simulink model "ES101A_DiagcMgr"  (R2013b)
settings: Solver=ode45  StartTime=0.0  StopTime=0.44  RelTol=1e-3
values from neighbouring files (symbols this model uses):
  BrdgVltg = DataDict.IpSignal    [ES101A_DiagcMgr_DataDict.m]
  DEM_CLEAR_PENDING = DataDict.Constant    [ES101A_DiagcMgr_DataDict.m]
  DEM_DTC_GROUP_ALL_DTCS = DataDict.Constant    [ES101A_DiagcMgr_DataDict.m]
  DFTAGICNTR_CNT_U08 = DataDict.Constant    [ES101A_DiagcMgr_DataDict.m]
  DIAGCMGR_NTCINFOSTSTESTFAILD_CNT_U08 = DataDict.Constant    [ES101A_DiagcMgr_DataDict.m]
  DIAGCMGR_NTCINFOSTSTESTFAILDTHISIGNCYC_CNT_U08 = DataDict.Constant    [ES101A_DiagcMgr_DataDict.m]
  DIAGCMGR_NTCINFOSTSTESTNOTCMPLTHISIGNCYC_CNT_U08 = DataDict.Constant    [ES101A_DiagcMgr_DataDict.m]
  DiagcMgrFltResp = DataDict.Calibration    [ES101A_DiagcMgr_DataDict.m]
  DiagcMgrNtcFltAry = DataDict.NVM    [ES101A_DiagcMgr_DataDict.m]
  DIAGCSTSCTRLDSHTDWNFLTPRSNT_CNT_U16 = DataDict.Constant    [ES101A_DiagcMgr_DataDict.m]
  DIAGCSTSDFTHWAG_CNT_U16 = DataDict.Constant    [ES101A_DiagcMgr_DataDict.m]
  DIAGCSTSDFTHWAGSERLCOMEXPRTVAL_CNT_U16 = DataDict.Constant    [ES101A_DiagcMgr_DataDict.m]
  DIAGCSTSDFTVEHSPD_CNT_U16 = DataDict.Constant    [ES101A_DiagcMgr_DataDict.m]
  DIAGCSTSININVAL_CNT_U16 = DataDict.Constant    [ES101A_DiagcMgr_DataDict.m]
  DIAGCSTSIVTR1INACTV_CNT_U16 = DataDict.Constant    [ES101A_DiagcMgr_DataDict.m]
  DIAGCSTSIVTR2INACTV_CNT_U16 = DataDict.Constant    [ES101A_DiagcMgr_DataDict.m]
  DIAGCSTSLIMDTPRFMNC_CNT_U16 = DataDict.Constant    [ES101A_DiagcMgr_DataDict.m]
  DIAGCSTSRAMPTOZEROFLTPRSNT_CNT_U16 = DataDict.Constant    [ES101A_DiagcMgr_DataDict.m]
  DIAGCSTSWHLIMBREJCTNDI_CNT_U16 = DataDict.Constant    [ES101A_DiagcMgr_DataDict.m]
  DTCIDXSTSFAIL_CNT_U08 = DataDict.Constant    [ES101A_DiagcMgr_DataDict.m]
  DTCIDXSTSNONTC_CNT_U08 = DataDict.Constant    [ES101A_DiagcMgr_DataDict.m]
  DTCIDXSTSNORES_CNT_U08 = DataDict.Constant    [ES101A_DiagcMgr_DataDict.m]
  DTCIDXSTSPASS_CNT_U08 = DataDict.Constant    [ES101A_DiagcMgr_DataDict.m]
  DTCIDXSTSUPDCFMD_CNT_U08 = DataDict.Constant    [ES101A_DiagcMgr_DataDict.m]
  ELECGLBPRM_IVTRCNT_CNT_U08 = DataDict.ConfigParam    [ES101A_DiagcMgr_DataDict.m]
  FLTINJ_DIAGCMGR_DIAGCSTSIVTR1INACTV = DataDict.Constant    [ES101A_DiagcMgr_DataDict.m]
  FLTINJ_DIAGCMGR_DIAGCSTSIVTR2INACTV = DataDict.Constant    [ES101A_DiagcMgr_DataDict.m]
  HwTq = DataDict.IpSignal    [ES101A_DiagcMgr_DataDict.m]
  IgnCntr = DataDict.IpSignal    [ES101A_DiagcMgr_DataDict.m]
  MAXDEBCNTRVAL_CNT_S16 = DataDict.Constant    [ES101A_DiagcMgr_DataDict.m]
  MAXRAMPRATE_ULSPERSEC_F32 = DataDict.Constant    [ES101A_DiagcMgr_DataDict.m]
  MINDEBCNTRVAL_CNT_S16 = DataDict.Constant    [ES101A_DiagcMgr_DataDict.m]
  MINRAMPRATE_ULSPERSEC_F32 = DataDict.Constant    [ES101A_DiagcMgr_DataDict.m]
  SCAMOTTQCMDTOONE_ULS_F32 = DataDict.Constant    [ES101A_DiagcMgr_DataDict.m]
  SCAMOTTQCMDTOZERO_ULS_F32 = DataDict.Constant    [ES101A_DiagcMgr_DataDict.m]
  SysSt = DataDict.IpSignal    [ES101A_DiagcMgr_DataDict.m]
  VehSpd = DataDict.IpSignal    [ES101A_DiagcMgr_DataDict.m]
undefined symbols (not defined in the file or in its folder): ActvMotTqCmdSca, ActvRampRate, AgiCntr, Dem_DTCFormatType, Dem_DTCOriginType, Dem_EventStatusType, DiagcData, DiagcMgrNtcMap, DiagcSts, DtcEnaMask, EcuT, HistNtcFltAry, MicroDiagcData, MotTq, NtcNr, NtcNrWithResd1, NtcStInfo, ProxySetNtcData, Sts, SysSt1, TOTNROFDTC_CNT_U08
libraries: simulink x151, FloatToFixd x5, NxtrNvM x4
(part 3 of 13)

== system ES101A_DiagcMgr/DiagcMgr/ClrAllDiagc/If Action Subsystem1 ==
  Action Port : ActionPort  ActionType=else
  Set : Constant
  ClrDiagcFlg : Outport
  wires:
  Set/1 -> ClrDiagcFlg/1

== system ES101A_DiagcMgr/DiagcMgr/ClrSnpshtData/CopyRight2 ==

== system ES101A_DiagcMgr/DiagcMgr/ClrSnpshtData/Subsystem ==
  Length of Snapshot Array : Inport
  Assignment1 : Assignment  IndexMode=Zero-based  IndexOptions=Index vector (port)  Indices=1  OutputSizes=1
  Bus Assignment3 : BusAssignment  AssignedSignals=MicroDiagcData,HwTq,MotTq,IgnCntr,BrdgVltg,EcuT,NtcNr,NtcStInfo,SysSt,VehSpd
  Constant1 : Constant  Value=0  OutDataTypeStr=uint32
  Constant12 : Constant  Value=0  OutDataTypeStr=uint8
  Constant{2..4,7..8} (5 alike) : Constant  Value=0  OutDataTypeStr=single
  Constant5 : Constant  Value=SysSt1.SYSST_WRMININ  OutDataTypeStr=Enum: SysSt1
  Constant6 : Constant  Value=0  OutDataTypeStr=uint32
  Constant9 : Constant  Value=NtcNrWithResd1.NTCNR_RESD  OutDataTypeStr=Enum: NtcNrWithResd1
  CopyRight2 : Subsystem  Description=|  mask(Copyright Information){none=on}
      | Copyright info block.                                               
      |                                                                     
      | Place copyright information at the top of every subsystem in design.
      mask prompts: none "No parameters"
      mask help: Place copyright information at the top of every subsystem in design.
      mask Display:
      | NxtrConf = 'Nexteer Confidential';
      | 
      | sys = bdroot; %handle for the current model ("system")
      | first = get_param(sys,'Created');
      | first = first(end-3:end);  %year is last four digits
      | 
      | last = get_param(sys,'LastModifiedDate');
      | if isempty(last)
      |     last = datestr(now,'yyyy');
      | else
      |     last = last(end-3:end);
      | end
      | 
      | if strcmp(first,last)
      |     fprintf('%s -- Copyright %s Nexteer',NxtrConf,first)
      | else
      |     fprintf('%s -- %s%s- %s Nexteer',NxtrConf,char(169),first,last)
      | end
  Data Store Read1 : DataStoreRead  DataStoreName=SnpshtDataAry
  Data Store Write2 : DataStoreWrite  DataStoreName=SnpshtDataAry
  For Iterator : ForIterator  IterationSource=external  IndexMode=Zero-based
  Selector1 : Selector  IndexMode=Zero-based  InputPortWidth=20  IndexOptions=Index vector (port)  Indices=[1 3]  OutputSizes=1
  wires:
  Length of Snapshot Array/1 -> For Iterator/1
  For Iterator/1 -> Selector1/2, Assignment1/3
  Bus Assignment3/1 -> Assignment1/2
  Assignment1/1 -> Data Store Write2/1
  Selector1/1 -> Bus Assignment3/1
  Data Store Read1/1 -> Selector1/1, Assignment1/1
  Constant9/1 -> Bus Assignment3/8
  Constant5/1 -> Bus Assignment3/10
  Constant12/1 -> Bus Assignment3/9
  Constant6/1 -> Bus Assignment3/5
  Constant3/1 -> Bus Assignment3/4
  Constant2/1 -> Bus Assignment3/3
  Constant4/1 -> Bus Assignment3/11
  Constant8/1 -> Bus Assignment3/7
  Constant1/1 -> Bus Assignment3/2
  Constant7/1 -> Bus Assignment3/6

== system ES101A_DiagcMgr/DiagcMgr/DiagcMgrIninCore/CopyRight2 ==

== system ES101A_DiagcMgr/DiagcMgr/DiagcMgrIninCore/Initialize the NtcInfo Array ==
  NtcInfoArySize : Inport
  NtcInfoAry_ArgIn : Inport  Port=2
  CopyRight2 : Subsystem  Description=|  mask(Copyright Information){none=on}
      | Copyright info block.                                               
      |                                                                     
      | Place copyright information at the top of every subsystem in design.
      mask prompts: none "No parameters"
      mask help: Place copyright information at the top of every subsystem in design.
      mask Display:
      | NxtrConf = 'Nexteer Confidential';
      | 
      | sys = bdroot; %handle for the current model ("system")
      | first = get_param(sys,'Created');
      | first = first(end-3:end);  %year is last four digits
      | 
      | last = get_param(sys,'LastModifiedDate');
      | if isempty(last)
      |     last = datestr(now,'yyyy');
      | else
      |     last = last(end-3:end);
      | end
      | 
      | if strcmp(first,last)
      |     fprintf('%s -- Copyright %s Nexteer',NxtrConf,first)
      | else
      |     fprintf('%s -- %s%s- %s Nexteer',NxtrConf,char(169),first,last)
      | end
  Update the ISO bits of each NTC : Subsystem  RequirementInfo={} %GIDa_598903a9_4093_4047_8f55_d30b0bb8de3e  Priority=2  TreatAsAtomicUnit=on
      settings: AttributesFormatString=Priority = %<Priority>
  NtcInfoAry_ArgOut : Outport
  wires:
  NtcInfoArySize/1 -> Update the ISO bits of each NTC/1(Number of Iteration)
  Update the ISO bits of each NTC/1(NtcInfoAry_ArgOut) -> NtcInfoAry_ArgOut/1
  NtcInfoAry_ArgIn/1 -> Update the ISO bits of each NTC/2(NtcInfoAry_ArgIn)

== system ES101A_DiagcMgr/DiagcMgr/DiagcMgrIninCore/Update DiagcSts and DiagcMgrActv ==
  note: ProxySetNtcData and DiagcData are inputs to the port "Bus"
      | of the Bus Assignment Block are not inputs, outputs or arguments to the
      | DiagcMgrIninCore. They are being used for modelling purpose to show
      | that the data is being written to the respective structs.
  ProxySetNtcData : Inport
  DiagcData : Inport  Port=2
  Bus Assignment1 : BusAssignment  AssignedSignals=DiagcSts,ActvRampRate,ActvMotTqCmdSca
  Bus Assignment2 : BusAssignment  AssignedSignals=DiagcSts,ActvRampRate,ActvMotTqCmdSca
  CopyRight2 : Subsystem  Description=|  mask(Copyright Information){none=on}
      | Copyright info block.                                               
      |                                                                     
      | Place copyright information at the top of every subsystem in design.
      mask prompts: none "No parameters"
      mask help: Place copyright information at the top of every subsystem in design.
      mask Display:
      | NxtrConf = 'Nexteer Confidential';
      | 
      | sys = bdroot; %handle for the current model ("system")
      | first = get_param(sys,'Created');
      | first = first(end-3:end);  %year is last four digits
      | 
      | last = get_param(sys,'LastModifiedDate');
      | if isempty(last)
      |     last = datestr(now,'yyyy');
      | else
      |     last = last(end-3:end);
      | end
      | 
      | if strcmp(first,last)
      |     fprintf('%s -- Copyright %s Nexteer',NxtrConf,first)
      | else
      |     fprintf('%s -- %s%s- %s Nexteer',NxtrConf,char(169),first,last)
      | end
  DiagcStsActvMotTqCmdSca : Constant  Value=SCAMOTTQCMDTOONE_ULS_F32  OutDataTypeStr=single
  DiagcStsActvRampRate : Constant  Value=MINRAMPRATE_ULSPERSEC_F32  OutDataTypeStr=single
  Dual Inverter : Subsystem  TreatAsAtomicUnit=on
  If1 : If  IfExpression=u1 == 1
  Merge : Merge
  Number of Inverters : Constant  Value=ELECGLBPRM_IVTRCNT_CNT_U08
  ProxySetNtcActvMotTqCmdSca : Constant  Value=SCAMOTTQCMDTOONE_ULS_F32  OutDataTypeStr=single
  ProxySetNtcActvRampRate : Constant  Value=MINRAMPRATE_ULSPERSEC_F32  OutDataTypeStr=single
  Single Inverter : Subsystem  Description=""  TreatAsAtomicUnit=on
      settings: AttributesFormatString=%<Description>
  ProxySetNtcData_ArgOut : Outport
  DiagcData_ArgOut : Outport  Port=2
  wires:
  Number of Inverters/1 -> If1/1
  If1/1 -> Single Inverter/Action
  ProxySetNtcActvMotTqCmdSca/1 -> Bus Assignment1/4
  ProxySetNtcActvRampRate/1 -> Bus Assignment1/3
  Bus Assignment1/1 -> ProxySetNtcData_ArgOut/1
  If1/2 -> Dual Inverter/Action
  Single Inverter/1(DiagcSts) -> Merge/1
  Dual Inverter/1(DiagcSts) -> Merge/2
  Merge/1 -> Bus Assignment2/2, Bus Assignment1/2
  Bus Assignment2/1 -> DiagcData_ArgOut/1
  DiagcStsActvRampRate/1 -> Bus Assignment2/3
  DiagcStsActvMotTqCmdSca/1 -> Bus Assignment2/4
  ProxySetNtcData/1 -> Bus Assignment1/1
  DiagcData/1 -> Bus Assignment2/1

== system ES101A_DiagcMgr/DiagcMgr/DiagcMgrIninCore/Update NtcInfoAry From NvM ==
  AppIdx_ArgIn : Inport
  NtcInfoAry_ArgIn : Inport  Port=2
  CopyRight2 : Subsystem  Description=|  mask(Copyright Information){none=on}
      | Copyright info block.                                               
      |                                                                     
      | Place copyright information at the top of every subsystem in design.
      mask prompts: none "No parameters"
      mask help: Place copyright information at the top of every subsystem in design.
      mask Display:
      | NxtrConf = 'Nexteer Confidential';
      | 
      | sys = bdroot; %handle for the current model ("system")
      | first = get_param(sys,'Created');
      | first = first(end-3:end);  %year is last four digits
      | 
      | last = get_param(sys,'LastModifiedDate');
      | if isempty(last)
      |     last = datestr(now,'yyyy');
      | else
      |     last = last(end-3:end);
      | end
      | 
      | if strcmp(first,last)
      |     fprintf('%s -- Copyright %s Nexteer',NxtrConf,first)
      | else
      |     fprintf('%s -- %s%s- %s Nexteer',NxtrConf,char(169),first,last)
      | end
  Data Store Read1 : DataStoreRead  DataStoreName=DiagcMgrNtcFltAry
  Update NtcInfoAry : Subsystem
  Width : Width  DataType=uint8
  NtcInfoAry_ArgOut : Outport
  wires:
  Width/1 -> Update NtcInfoAry/1(Length of NtcFltArray)
  AppIdx_ArgIn/1 -> Update NtcInfoAry/2(AppIdx_ArgIn)
  Data Store Read1/1 -> Width/1
  NtcInfoAry_ArgIn/1 -> Update NtcInfoAry/3(NtcInfoAry_ArgIn)
  Update NtcInfoAry/1(NtcInfoAry_ArgOut) -> NtcInfoAry_ArgOut/1

== system ES101A_DiagcMgr/DiagcMgr/DiagcMgrPer1/CopyRight2 ==

== system ES101A_DiagcMgr/DiagcMgr/DiagcMgrPer1/Update OutpDiagcData ==
  Bus Selector : BusSelector  OutputSignals=DiagcSts,ActvRampRate,ActvMotTqCmdSca
  CopyRight2 : Subsystem  Description=|  mask(Copyright Information){none=on}
      | Copyright info block.                                               
      |                                                                     
      | Place copyright information at the top of every subsystem in design.
      mask prompts: none "No parameters"
      mask help: Place copyright information at the top of every subsystem in design.
      mask Display:
      | NxtrConf = 'Nexteer Confidential';
      | 
      | sys = bdroot; %handle for the current model ("system")
      | first = get_param(sys,'Created');
      | first = first(end-3:end);  %year is last four digits
      | 
      | last = get_param(sys,'LastModifiedDate');
      | if isempty(last)
      |     last = datestr(now,'yyyy');
      | else
      |     last = last(end-3:end);
      | end
      | 
      | if strcmp(first,last)
      |     fprintf('%s -- Copyright %s Nexteer',NxtrConf,first)
      | else
      |     fprintf('%s -- %s%s- %s Nexteer',NxtrConf,char(169),first,last)
      | end
  GetDiagcDataApplX : Subsystem  RequirementInfo={} %GIDa_c222c484_d216_46ea_ad62_3550c5adb482
      settings: AttributesFormatString=%<Description>
  OutpDiagcSts : Outport
  OutpRampRate : Outport  Port=2
  OutpMotTqCmdSca : Outport  Port=3
  wires:
  Bus Selector/1 -> OutpDiagcSts/1  "<DiagcSts>"
  Bus Selector/3 -> OutpMotTqCmdSca/1  "<ActvMotTqCmdSca>"
  Bus Selector/2 -> OutpRampRate/1  "<ActvRampRate>"
  GetDiagcDataApplX/1(TempDiagcData) -> Bus Selector/1

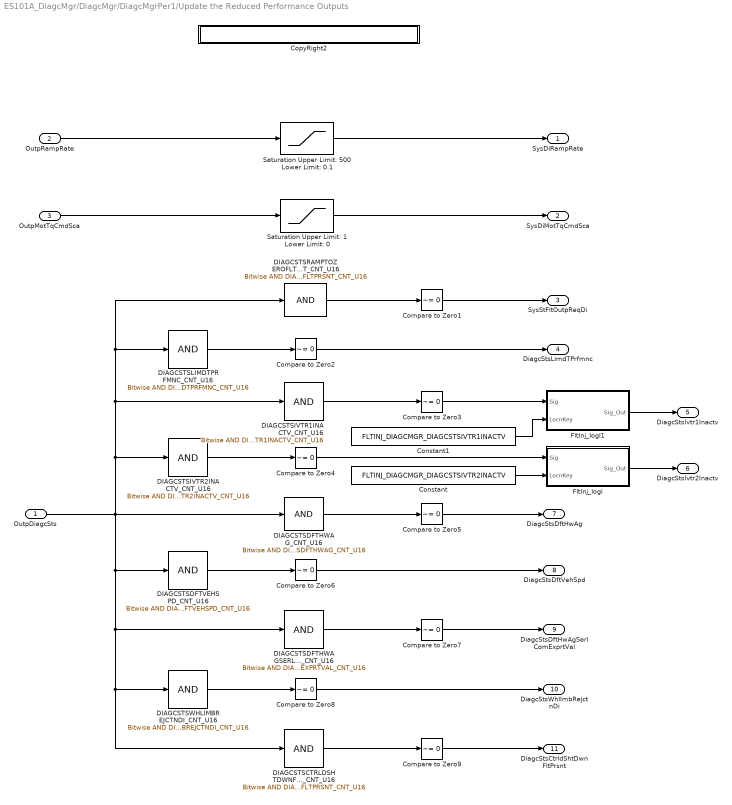
== system ES101A_DiagcMgr/DiagcMgr/DiagcMgrPer1/Update the Reduced Performance Outputs ==
  OutpDiagcSts : Inport
  OutpRampRate : Inport  Port=2
  OutpMotTqCmdSca : Inport  Port=3
  Compare to Zero{1..9} (9 alike) : simulink/Logic and Bit Operations/Compare To Zero  relop=~=  OutDataTypeStr=boolean
  Constant : Constant  Value=FLTINJ_DIAGCMGR_DIAGCSTSIVTR2INACTV
  Constant1 : Constant  Value=FLTINJ_DIAGCMGR_DIAGCSTSIVTR1INACTV
  CopyRight2 : Subsystem  Description=|  mask(Copyright Information){none=on}
      | Copyright info block.                                               
      |                                                                     
      | Place copyright information at the top of every subsystem in design.
      mask prompts: none "No parameters"
      mask help: Place copyright information at the top of every subsystem in design.
      mask Display:
      | NxtrConf = 'Nexteer Confidential';
      | 
      | sys = bdroot; %handle for the current model ("system")
      | first = get_param(sys,'Created');
      | first = first(end-3:end);  %year is last four digits
      | 
      | last = get_param(sys,'LastModifiedDate');
      | if isempty(last)
      |     last = datestr(now,'yyyy');
      | else
      |     last = last(end-3:end);
      | end
      | 
      | if strcmp(first,last)
      |     fprintf('%s -- Copyright %s Nexteer',NxtrConf,first)
      | else
      |     fprintf('%s -- %s%s- %s Nexteer',NxtrConf,char(169),first,last)
      | end
  DIAGCSTSCTRLDSHTDWNFLTPRSNT_CNT_U16 : simulink/Logic and Bit Operations/Bitwise Operator  logicop=AND  UseBitMask=on  BitMask=DIAGCSTSCTRLDSHTDWNFLTPRSNT_CNT_U16  BitMaskRealWorld=Stored Integer
  DIAGCSTSDFTHWAGSERLCOMEXPRTVAL_CNT_U16 : simulink/Logic and Bit Operations/Bitwise Operator  logicop=AND  UseBitMask=on  BitMask=DIAGCSTSDFTHWAGSERLCOMEXPRTVAL_CNT_U16  BitMaskRealWorld=Stored Integer
  DIAGCSTSDFTHWAG_CNT_U16 : simulink/Logic and Bit Operations/Bitwise Operator  logicop=AND  UseBitMask=on  BitMask=DIAGCSTSDFTHWAG_CNT_U16  BitMaskRealWorld=Stored Integer
  DIAGCSTSDFTVEHSPD_CNT_U16 : simulink/Logic and Bit Operations/Bitwise Operator  logicop=AND  UseBitMask=on  BitMask=DIAGCSTSDFTVEHSPD_CNT_U16  BitMaskRealWorld=Stored Integer
  DIAGCSTSIVTR1INACTV_CNT_U16 : simulink/Logic and Bit Operations/Bitwise Operator  logicop=AND  UseBitMask=on  BitMask=DIAGCSTSIVTR1INACTV_CNT_U16  BitMaskRealWorld=Stored Integer
  DIAGCSTSIVTR2INACTV_CNT_U16 : simulink/Logic and Bit Operations/Bitwise Operator  logicop=AND  UseBitMask=on  BitMask=DIAGCSTSIVTR2INACTV_CNT_U16  BitMaskRealWorld=Stored Integer
  DIAGCSTSLIMDTPRFMNC_CNT_U16 : simulink/Logic and Bit Operations/Bitwise Operator  logicop=AND  UseBitMask=on  BitMask=DIAGCSTSLIMDTPRFMNC_CNT_U16  BitMaskRealWorld=Stored Integer
  DIAGCSTSRAMPTOZEROFLTPRSNT_CNT_U16 : simulink/Logic and Bit Operations/Bitwise Operator  logicop=AND  UseBitMask=on  BitMask=DIAGCSTSRAMPTOZEROFLTPRSNT_CNT_U16  BitMaskRealWorld=Stored Integer
  DIAGCSTSWHLIMBREJCTNDI_CNT_U16 : simulink/Logic and Bit Operations/Bitwise Operator  logicop=AND  UseBitMask=on  BitMask=DIAGCSTSWHLIMBREJCTNDI_CNT_U16  BitMaskRealWorld=Stored Integer
  FltInj_logl : Subsystem  RequirementInfo="{'linktype_rmi_doors' '0000c474 (/ESG Group/FDD Module Requirements/EA4 Specific/ES101A_DiagcMgr)' '#ES101A_351' 'true' 'REQ:  ES101A_351' '' } %GIDa_b390188d_b896_424c_9f58_fe8516a642f6"  TreatAsAtomicUnit=on  VariantControl=FLTINJENA ~= STD_ON  mask(Fault_Injection){}
      mask help: Simulation mode is just a pass-thru.
  FltInj_logl1 : Subsystem  RequirementInfo="{'linktype_rmi_doors' '0000c474 (/ESG Group/FDD Module Requirements/EA4 Specific/ES101A_DiagcMgr)' '#ES101A_350' 'true' 'REQ:  ES101A_350' '' } %GIDa_e94889bb_00af_4b2c_a06f_23efdc67c67c"  TreatAsAtomicUnit=on  VariantControl=FLTINJENA ~= STD_ON  mask(Fault_Injection){}
      mask help: Simulation mode is just a pass-thru.
  Saturation Upper Limit: 1 Lower Limit: 0 : Saturate  UpperLimit=SCAMOTTQCMDTOONE_ULS_F32  LowerLimit=SCAMOTTQCMDTOZERO_ULS_F32
  Saturation Upper Limit: 500 Lower Limit: 0.1 : Saturate  UpperLimit=MAXRAMPRATE_ULSPERSEC_F32  LowerLimit=MINRAMPRATE_ULSPERSEC_F32
  SysDiRampRate : Outport
  SysDiMotTqCmdSca : Outport  Port=2  OutMin=[0]  OutMax=[1]  InitialOutput=1
  SysStFltOutpReqDi : Outport  Port=3
  DiagcStsLimdTPrfmnc : Outport  Port=4
  DiagcStsIvtr1Inactv : Outport  Port=5
  DiagcStsIvtr2Inactv : Outport  Port=6
  DiagcStsDftHwAg : Outport  RequirementInfo={} %GIDa_12676038_d59f_4b2e_bb2e_c1ecabcb392d  Port=7
  DiagcStsDftVehSpd : Outport  RequirementInfo={} %GIDa_cfb20322_9919_4223_82ea_8aaccca9938a  Port=8
  DiagcStsDftHwAgSerlComExprtVal : Outport  RequirementInfo={} %GIDa_a5c066d2_ac4d_4de0_aaf2_833db357af64  Port=9
  DiagcStsWhlImbRejctnDi : Outport  RequirementInfo={} %GIDa_3ef233f9_5c2f_4113_8632_848f684dd040  Port=10
  DiagcStsCtrldShtDwnFltPrsnt : Outport  RequirementInfo={} %GIDa_c67dadea_f274_4d61_964c_dd940fbe2d55  Port=11
  wires:
  OutpRampRate/1 -> Saturation Upper Limit: 500 Lower Limit: 0.1/1
  DIAGCSTSRAMPTOZEROFLTPRSNT_CNT_U16/1 -> Compare to Zero1/1
  Compare to Zero1/1 -> SysStFltOutpReqDi/1
  DIAGCSTSLIMDTPRFMNC_CNT_U16/1 -> Compare to Zero2/1
  Compare to Zero2/1 -> DiagcStsLimdTPrfmnc/1
  DIAGCSTSIVTR1INACTV_CNT_U16/1 -> Compare to Zero3/1
  DIAGCSTSIVTR2INACTV_CNT_U16/1 -> Compare to Zero4/1
  OutpMotTqCmdSca/1 -> Saturation Upper Limit: 1 Lower Limit: 0/1
  Compare to Zero5/1 -> DiagcStsDftHwAg/1
  Compare to Zero6/1 -> DiagcStsDftVehSpd/1
  Compare to Zero7/1 -> DiagcStsDftHwAgSerlComExprtVal/1
  Compare to Zero8/1 -> DiagcStsWhlImbRejctnDi/1
  DIAGCSTSDFTHWAG_CNT_U16/1 -> Compare to Zero5/1
  DIAGCSTSDFTVEHSPD_CNT_U16/1 -> Compare to Zero6/1
  DIAGCSTSDFTHWAGSERLCOMEXPRTVAL_CNT_U16/1 -> Compare to Zero7/1
  DIAGCSTSWHLIMBREJCTNDI_CNT_U16/1 -> Compare to Zero8/1
  OutpDiagcSts/1 -> DIAGCSTSCTRLDSHTDWNFLTPRSNT_CNT_U16/1, DIAGCSTSWHLIMBREJCTNDI_CNT_U16/1, DIAGCSTSDFTHWAGSERLCOMEXPRTVAL_CNT_U16/1, DIAGCSTSDFTVEHSPD_CNT_U16/1, DIAGCSTSIVTR1INACTV_CNT_U16/1, DIAGCSTSRAMPTOZEROFLTPRSNT_CNT_U16/1, DIAGCSTSLIMDTPRFMNC_CNT_U16/1, DIAGCSTSIVTR2INACTV_CNT_U16/1, DIAGCSTSDFTHWAG_CNT_U16/1
  Compare to Zero9/1 -> DiagcStsCtrldShtDwnFltPrsnt/1
  DIAGCSTSCTRLDSHTDWNFLTPRSNT_CNT_U16/1 -> Compare to Zero9/1
  Saturation Upper Limit: 500 Lower Limit: 0.1/1 -> SysDiRampRate/1
  Saturation Upper Limit: 1 Lower Limit: 0/1 -> SysDiMotTqCmdSca/1
  Compare to Zero4/1 -> FltInj_logl/1(Sig)
  FltInj_logl/1(Sig_Out) -> DiagcStsIvtr2Inactv/1
  Constant/1 -> FltInj_logl/2("LocnKey  ")
  FltInj_logl1/1(Sig_Out) -> DiagcStsIvtr1Inactv/1
  Compare to Zero3/1 -> FltInj_logl1/1(Sig)
  Constant1/1 -> FltInj_logl1/2("LocnKey  ")

== system ES101A_DiagcMgr/DiagcMgr/DiagcMgrPer2/Clear All DTCs ==
  note: NOTE:
      | 	In Periodic 2, the ClearDTC function is called multiple times based on the
      | 	return status of the ClearDTC. Initially, when we call the DEM with the argument
      | 	DEM_DTC_GROUP_ALL_DTCS to clear all DTCs, the DEM enters a locked state.
      | 	Any further calls to the DEM with any argument that is different from the ones last passed,
      | 	will return us a status of BUSY.
      | 	When the first request is made to clear all DTCs, the DEM returns PENDING Status if
      | 	DTCs haven't been cleared yet.	The main function in DEM which runs at 10ms clears the
      | 	DTCs. Once the DTCs are cleared,
      | 	if a call is made to the DEM with the same parameters as before, E_OK is returned.
      | 	We stop calling the DEM with the DEM_DTC_GROUP_ALL_DTCS once we receive any
      | 	other status apart from PENDING.
  Action Port : ActionPort
  Call DEM & Update DtcIdxPrevSts : Subsystem
  CopyRight2 : Subsystem  Description=|  mask(Copyright Information){none=on}
      | Copyright info block.                                               
      |                                                                     
      | Place copyright information at the top of every subsystem in design.
      mask prompts: none "No parameters"
      mask help: Place copyright information at the top of every subsystem in design.
      mask Display:
      | NxtrConf = 'Nexteer Confidential';
      | 
      | sys = bdroot; %handle for the current model ("system")
      | first = get_param(sys,'Created');
      | first = first(end-3:end);  %year is last four digits
      | 
      | last = get_param(sys,'LastModifiedDate');
      | if isempty(last)
      |     last = datestr(now,'yyyy');
      | else
      |     last = last(end-3:end);
      | end
      | 
      | if strcmp(first,last)
      |     fprintf('%s -- Copyright %s Nexteer',NxtrConf,first)
      | else
      |     fprintf('%s -- %s%s- %s Nexteer',NxtrConf,char(169),first,last)
      | end

== system ES101A_DiagcMgr/DiagcMgr/DiagcMgrPer2/CopyRight2 ==

== system ES101A_DiagcMgr/DiagcMgr/DiagcMgrPer2/Normal Periodic Processing ==
  note: An array of Temp Variable, DtcIdxCurrSts (DTC Index Current Status)
      | 	Properties:
      | 		Variable Length for each build/program depending on the Number of DTCs for that program.
      | 		Data is subject to change based on respective linked NTC Status
      | 		Length of the Array is TOTNROFDTC_CNT_U08 + 1.
      |
      |
      | 	DtcIdxPrevSts Bit Info:
      | 		Bit [0:1]:
      | 		0 No Result
      | 		1 Pass
      | 		2 Fail
      | 		3 No NTC
      |
      | 		Bit [2:7]:
      | 		Reserved
  Action Port : ActionPort  ActionType=else
  CopyRight2 : Subsystem  Description=|  mask(Copyright Information){none=on}
      | Copyright info block.                                               
      |                                                                     
      | Place copyright information at the top of every subsystem in design.
      mask prompts: none "No parameters"
      mask help: Place copyright information at the top of every subsystem in design.
      mask Display:
      | NxtrConf = 'Nexteer Confidential';
      | 
      | sys = bdroot; %handle for the current model ("system")
      | first = get_param(sys,'Created');
      | first = first(end-3:end);  %year is last four digits
      | 
      | last = get_param(sys,'LastModifiedDate');
      | if isempty(last)
      |     last = datestr(now,'yyyy');
      | else
      |     last = last(end-3:end);
      | end
      | 
      | if strcmp(first,last)
      |     fprintf('%s -- Copyright %s Nexteer',NxtrConf,first)
      | else
      |     fprintf('%s -- %s%s- %s Nexteer',NxtrConf,char(169),first,last)
      | end
  For All DTCs : Subsystem  RequirementInfo="{'linktype_rmi_doors' '0000c474 (/ESG Group/FDD Module Requirements/EA4 Specific/ES101A_DiagcMgr)' '#ES101A_311' 'true' 'REQ:  ES101A_311' '' ; 'linktype_rmi_doors' '0000c474 (/ESG Group/FDD Module Requirements/EA4 Specific/ES101A_DiagcMgr)' '#ES101A_312' 'true' 'REQ:  ES101A_312' '' ; 'linktype_rmi_doors' '0000c474 (/ESG Group/FDD Module Requirements/EA4 Specific/ES101A_DiagcMgr)' '#ES101A_314' 'true' 'REQ:  ES101A_314' '' } %GIDa_9b82b52b_93f6_4b1b_ba3f_eb413fcb8afc"  Priority=3  TreatAsAtomicUnit=on
      settings: AttributesFormatString=Priority = %<Priority>
  For All NTCs : Subsystem  Priority=2  TreatAsAtomicUnit=on
      settings: AttributesFormatString=Priority = %<Priority>
  Initialize DtcIdxCurrSts : Subsystem  Priority=1  TreatAsAtomicUnit=on
      settings: AttributesFormatString=Priority = %<Priority>
  TempVar: DTC Index Current Status : DataStoreMemory  Description=|  DataStoreName=DtcIdxCurrSts  OutDataTypeStr=uint16  StateMustResolveToSignalObject=on
      | All Elements of this array should be
      | initialized to 0x03 everytime we enter DiagcMgrPer2
      settings: AttributesFormatString=%<Description>

== system ES101A_DiagcMgr/DiagcMgr/DiagcMgrPwrDwn/Clear NtcFltAryIdx and HistFltAryIdx ==
  CopyRight2 : Subsystem  Description=|  mask(Copyright Information){none=on}
      | Copyright info block.                                               
      |                                                                     
      | Place copyright information at the top of every subsystem in design.
      mask prompts: none "No parameters"
      mask help: Place copyright information at the top of every subsystem in design.
      mask Display:
      | NxtrConf = 'Nexteer Confidential';
      | 
      | sys = bdroot; %handle for the current model ("system")
      | first = get_param(sys,'Created');
      | first = first(end-3:end);  %year is last four digits
      | 
      | last = get_param(sys,'LastModifiedDate');
      | if isempty(last)
      |     last = datestr(now,'yyyy');
      | else
      |     last = last(end-3:end);
      | end
      | 
      | if strcmp(first,last)
      |     fprintf('%s -- Copyright %s Nexteer',NxtrConf,first)
      | else
      |     fprintf('%s -- %s%s- %s Nexteer',NxtrConf,char(169),first,last)
      | end
  Data Store Write : DataStoreWrite  DataStoreName=NtcFltAryIdx  DataStoreElements=NtcFltAryIdx
  Data Store Write1 : DataStoreWrite  DataStoreName=HistFltAryIdx
  Data Store Write2 : DataStoreWrite  DataStoreName=NtcMapIdx
  Data Store Write3 : DataStoreWrite  DataStoreName=HistFltAryTempIdx
  Initial Value : Constant  OutDataTypeStr=uint8
  Length(HistFltAry) : Constant  Value=0  OutDataTypeStr=uint8
  Length(HistFltAry)1 : Constant  Value=0  OutDataTypeStr=uint8
  Length(NtcFltAry) : Constant  Value=0  OutDataTypeStr=uint8
  wires:
  Length(NtcFltAry)/1 -> Data Store Write/1
  Length(HistFltAry)/1 -> Data Store Write1/1
  Initial Value/1 -> Data Store Write2/1
  Length(HistFltAry)1/1 -> Data Store Write3/1

== system ES101A_DiagcMgr/DiagcMgr/DiagcMgrPwrDwn/CopyRight1 ==

== system ES101A_DiagcMgr/DiagcMgr/DiagcMgrPwrDwn/Update NtcFltAry and HistFltAry ==
  IC : Inport
  Add : Sum
  Bus Selector1 : BusSelector  OutputSignals=ApplIdx,NtcInfoIdx
  Compare To Constant : simulink/Logic and Bit Operations/Compare To Constant  relop=<=  const=20  OutDataTypeStr=boolean
  Compare To Constant1 : simulink/Logic and Bit Operations/Compare To Constant  relop=<=  const=511  OutDataTypeStr=boolean
  Constant : Constant  OutDataTypeStr=uint8
  CopyRight2 : Subsystem  Description=|  mask(Copyright Information){none=on}
      | Copyright info block.                                               
      |                                                                     
      | Place copyright information at the top of every subsystem in design.
      mask prompts: none "No parameters"
      mask help: Place copyright information at the top of every subsystem in design.
      mask Display:
      | NxtrConf = 'Nexteer Confidential';
      | 
      | sys = bdroot; %handle for the current model ("system")
      | first = get_param(sys,'Created');
      | first = first(end-3:end);  %year is last four digits
      | 
      | last = get_param(sys,'LastModifiedDate');
      | if isempty(last)
      |     last = datestr(now,'yyyy');
      | else
      |     last = last(end-3:end);
      | end
      | 
      | if strcmp(first,last)
      |     fprintf('%s -- Copyright %s Nexteer',NxtrConf,first)
      | else
      |     fprintf('%s -- %s%s- %s Nexteer',NxtrConf,char(169),first,last)
      | end
  Data Store Read1 : DataStoreRead  DataStoreName=NtcMapIdx  DataStoreElements=NtcMapIdx
  Data Store Read2 : DataStoreRead  DataStoreName=DiagcMgrNtcMap  DataStoreElements=DiagcMgrNtcMap(:)
  Data Store Read3 : DataStoreRead  DataStoreName=NtcFltAryIdx
  Data Store Read4 : DataStoreRead  DataStoreName=NtcMapIdx
  Data Store Write1 : DataStoreWrite  DataStoreName=NtcMapIdx
  For Number of NTCs : Subsystem  TreatAsAtomicUnit=on
  Logical Operator : Logic  AllPortsSameDT=off  OutDataTypeStr=boolean
  Selector1 : Selector  IndexMode=Zero-based  InputPortWidth=512  IndexOptions=Index vector (port)  Indices=[1 3]  OutputSizes=1
  While Iterator : WhileIterator  MaxIters=511  ShowIterationPort=on
  wires:
  Data Store Read2/1 -> Selector1/1
  Selector1/1 -> Bus Selector1/1
  While Iterator/1 -> For Number of NTCs/3(NtcMapIdx), Selector1/2
  Bus Selector1/1 -> For Number of NTCs/1(ApplIdx)  "<ApplIdx>"
  Bus Selector1/2 -> For Number of NTCs/2(NtcInfoIdx)  "<NtcInfoIdx>"
  IC/1 -> While Iterator/2
  Logical Operator/1 -> While Iterator/1
  Add/1 -> Data Store Write1/1
  Constant/1 -> Add/2
  Data Store Read1/1 -> Add/1
  Data Store Read3/1 -> Compare To Constant/1
  Compare To Constant/1 -> Logical Operator/1
  Compare To Constant1/1 -> Logical Operator/2
  Data Store Read4/1 -> Compare To Constant1/1

== system ES101A_DiagcMgr/DiagcMgr/DiagcMgrPwrDwn/While((HistFltAryTempIdx < HistFltInfoIdx) AND (NtcFltAryIdx < 20)) ==
  IC : Inport
  Add : Sum  Inputs=+-
  Compare To Constant1 : simulink/Logic and Bit Operations/Compare To Constant  relop=<  const=0  OutDataTypeStr=boolean
  Compare To Constant3 : simulink/Logic and Bit Operations/Compare To Constant  relop=<=  const=20  OutDataTypeStr=boolean
  CopyRight1 : Subsystem  Description=|  mask(Copyright Information){none=on}
      | Copyright info block.                                               
      |                                                                     
      | Place copyright information at the top of every subsystem in design.
      mask prompts: none "No parameters"
      mask help: Place copyright information at the top of every subsystem in design.
      mask Display:
      | NxtrConf = 'Nexteer Confidential';
      | 
      | sys = bdroot; %handle for the current model ("system")
      | first = get_param(sys,'Created');
      | first = first(end-3:end);  %year is last four digits
      | 
      | last = get_param(sys,'LastModifiedDate');
      | if isempty(last)
      |     last = datestr(now,'yyyy');
      | else
      |     last = last(end-3:end);
      | end
      | 
      | if strcmp(first,last)
      |     fprintf('%s -- Copyright %s Nexteer',NxtrConf,first)
      | else
      |     fprintf('%s -- %s%s- %s Nexteer',NxtrConf,char(169),first,last)
      | end
  Data Store Read2 : DataStoreRead  DataStoreName=HistFltAryIdx
  Data Store Read5 : DataStoreRead  DataStoreName=NtcFltAryIdx
  Data Store Read6 : DataStoreRead  DataStoreName=HistFltAryTempIdx
  Increment HistFltAryTempIdx and NtcFltAryIdx : Subsystem  Priority=2
      settings: AttributesFormatString=Priority = %<Priority>
  Logical Operator1 : Logic  AllPortsSameDT=off  OutDataTypeStr=boolean
  Update NtcFltAry : Subsystem  Priority=1
      settings: AttributesFormatString=|
      | Priority = %<Priority>
      | %<Description>
  While Iterator : WhileIterator  MaxIters=20  ResetStates=reset
  wires:
  Logical Operator1/1 -> While Iterator/1
  IC/1 -> While Iterator/2
  Data Store Read6/1 -> Add/1
  Data Store Read2/1 -> Add/2
  Add/1 -> Compare To Constant1/1
  Data Store Read5/1 -> Compare To Constant3/1
  Compare To Constant3/1 -> Logical Operator1/1
  Compare To Constant1/1 -> Logical Operator1/2

== system ES101A_DiagcMgr/DiagcMgr/DiagcMgrPwrDwn/While(CurrentFltIdx < TableSize[NtcFltAry]) ==
  IC : Inport
  Compare To Constant2 : simulink/Logic and Bit Operations/Compare To Constant  relop=<  const=20  OutDataTypeStr=boolean
  CopyRight1 : Subsystem  Description=|  mask(Copyright Information){none=on}
      | Copyright info block.                                               
      |                                                                     
      | Place copyright information at the top of every subsystem in design.
      mask prompts: none "No parameters"
      mask help: Place copyright information at the top of every subsystem in design.
      mask Display:
      | NxtrConf = 'Nexteer Confidential';
      | 
      | sys = bdroot; %handle for the current model ("system")
      | first = get_param(sys,'Created');
      | first = first(end-3:end);  %year is last four digits
      | 
      | last = get_param(sys,'LastModifiedDate');
      | if isempty(last)
      |     last = datestr(now,'yyyy');
      | else
      |     last = last(end-3:end);
      | end
      | 
      | if strcmp(first,last)
      |     fprintf('%s -- Copyright %s Nexteer',NxtrConf,first)
      | else
      |     fprintf('%s -- %s%s- %s Nexteer',NxtrConf,char(169),first,last)
      | end
  Data Store Read6 : DataStoreRead  DataStoreName=NtcFltAryIdx
  Increment Indices : Subsystem  Priority=2
      settings: AttributesFormatString=Priority = %<Priority>
  Update NtcFltAry : Subsystem  Priority=1
      settings: AttributesFormatString=Priority = %<Priority>
  While Iterator : WhileIterator  MaxIters=20
  wires:
  IC/1 -> While Iterator/2
  Data Store Read6/1 -> Compare To Constant2/1
  Compare To Constant2/1 -> While Iterator/1

== system ES101A_DiagcMgr/DiagcMgr/DiagcMgrPwrDwn/Write to NvM ==
  Constant1 : Constant  OutDataTypeStr=uint8
  CopyRight2 : Subsystem  Description=|  mask(Copyright Information){none=on}
      | Copyright info block.                                               
      |                                                                     
      | Place copyright information at the top of every subsystem in design.
      mask prompts: none "No parameters"
      mask help: Place copyright information at the top of every subsystem in design.
      mask Display:
      | NxtrConf = 'Nexteer Confidential';
      | 
      | sys = bdroot; %handle for the current model ("system")
      | first = get_param(sys,'Created');
      | first = first(end-3:end);  %year is last four digits
      | 
      | last = get_param(sys,'LastModifiedDate');
      | if isempty(last)
      |     last = datestr(now,'yyyy');
      | else
      |     last = last(end-3:end);
      | end
      | 
      | if strcmp(first,last)
      |     fprintf('%s -- Copyright %s Nexteer',NxtrConf,first)
      | else
      |     fprintf('%s -- %s%s- %s Nexteer',NxtrConf,char(169),first,last)
      | end
  Set Ram Block Status : NxtrNvM/Set Ram Block Status  FuncName=Set Ram Block Status  NvMBlockName=DiagcMgrNtcFltAry  VoidFuncRtn=on  BlockChanged_DSN=NvMSRBS_BlockChanged  Return_DSN=NvMSRBS_Return
      settings: AttributesFormatString=%<FuncName>
  wires:
  Constant1/1 -> Set Ram Block Status/1

== system ES101A_DiagcMgr/DiagcMgr/GetNtcActvCore /CopyRight2 ==

== system ES101A_DiagcMgr/DiagcMgr/GetNtcActvCore /GetNtcInfoAppIX ==
  NtcInfoIdx_ArgIn : Inport
  Action Port : ActionPort
  CopyRight2 : Subsystem  Description=|  mask(Copyright Information){none=on}
      | Copyright info block.                                               
      |                                                                     
      | Place copyright information at the top of every subsystem in design.
      mask prompts: none "No parameters"
      mask help: Place copyright information at the top of every subsystem in design.
      mask Display:
      | NxtrConf = 'Nexteer Confidential';
      | 
      | sys = bdroot; %handle for the current model ("system")
      | first = get_param(sys,'Created');
      | first = first(end-3:end);  %year is last four digits
      | 
      | last = get_param(sys,'LastModifiedDate');
      | if isempty(last)
      |     last = datestr(now,'yyyy');
      | else
      |     last = last(end-3:end);
      | end
      | 
      | if strcmp(first,last)
      |     fprintf('%s -- Copyright %s Nexteer',NxtrConf,first)
      | else
      |     fprintf('%s -- %s%s- %s Nexteer',NxtrConf,char(169),first,last)
      | end
  Data Store Read : DataStoreRead  DataStoreName=DiagcMgrNtcInfoX
  Selector : Selector  IndexMode=Zero-based  InputPortWidth=14  IndexOptions=Index vector (port)  Indices=[1 3]  OutputSizes=1
  NtcInfo_ArgOut : Outport
  wires:
  Data Store Read/1 -> Selector/1
  NtcInfoIdx_ArgIn/1 -> Selector/2
  Selector/1 -> NtcInfo_ArgOut/1

== system ES101A_DiagcMgr/DiagcMgr/GetNtcActvCore /NTC Not Active ==
  Action Port : ActionPort  ActionType=default
  Constant : Constant  Value=DIAGCMGR_NTCINFOSTSTESTNOTCMPLTHISIGNCYC_CNT_U08  OutDataTypeStr=uint8
  CopyRight2 : Subsystem  Description=|  mask(Copyright Information){none=on}
      | Copyright info block.                                               
      |                                                                     
      | Place copyright information at the top of every subsystem in design.
      mask prompts: none "No parameters"
      mask help: Place copyright information at the top of every subsystem in design.
      mask Display:
      | NxtrConf = 'Nexteer Confidential';
      | 
      | sys = bdroot; %handle for the current model ("system")
      | first = get_param(sys,'Created');
      | first = first(end-3:end);  %year is last four digits
      | 
      | last = get_param(sys,'LastModifiedDate');
      | if isempty(last)
      |     last = datestr(now,'yyyy');
      | else
      |     last = last(end-3:end);
      | end
      | 
      | if strcmp(first,last)
      |     fprintf('%s -- Copyright %s Nexteer',NxtrConf,first)
      | else
      |     fprintf('%s -- %s%s- %s Nexteer',NxtrConf,char(169),first,last)
      | end
  Sts : Outport
  wires:
  Constant/1 -> Sts/1

== system ES101A_DiagcMgr/DiagcMgr/GetNtcQlfrStsCore /CopyRight2 ==

== system ES101A_DiagcMgr/DiagcMgr/GetNtcQlfrStsCore /GetNtcInfoAppIX ==
  NtcInfoIdx_ArgIn : Inport
  Action Port : ActionPort
  CopyRight2 : Subsystem  Description=|  mask(Copyright Information){none=on}
      | Copyright info block.                                               
      |                                                                     
      | Place copyright information at the top of every subsystem in design.
      mask prompts: none "No parameters"
      mask help: Place copyright information at the top of every subsystem in design.
      mask Display:
      | NxtrConf = 'Nexteer Confidential';
      | 
      | sys = bdroot; %handle for the current model ("system")
      | first = get_param(sys,'Created');
      | first = first(end-3:end);  %year is last four digits
      | 
      | last = get_param(sys,'LastModifiedDate');
      | if isempty(last)
      |     last = datestr(now,'yyyy');
      | else
      |     last = last(end-3:end);
      | end
      | 
      | if strcmp(first,last)
      |     fprintf('%s -- Copyright %s Nexteer',NxtrConf,first)
      | else
      |     fprintf('%s -- %s%s- %s Nexteer',NxtrConf,char(169),first,last)
      | end
  Data Store Read : DataStoreRead  DataStoreName=DiagcMgrNtcInfoX
  Selector : Selector  IndexMode=Zero-based  InputPortWidth=14  IndexOptions=Index vector (port)  Indices=[1 3]  OutputSizes=1
  NtcInfo_ArgOut : Outport
  wires:
  Data Store Read/1 -> Selector/1
  NtcInfoIdx_ArgIn/1 -> Selector/2
  Selector/1 -> NtcInfo_ArgOut/1

== system ES101A_DiagcMgr/DiagcMgr/GetNtcQlfrStsCore /No Result State ==
  Action Port : ActionPort
  Constant : Constant  Value=DIAGCMGR_NTCINFOSTSTESTNOTCMPLTHISIGNCYC_CNT_U08  OutDataTypeStr=uint8
  CopyRight2 : Subsystem  Description=|  mask(Copyright Information){none=on}
      | Copyright info block.                                               
      |                                                                     
      | Place copyright information at the top of every subsystem in design.
      mask prompts: none "No parameters"
      mask help: Place copyright information at the top of every subsystem in design.
      mask Display:
      | NxtrConf = 'Nexteer Confidential';
      | 
      | sys = bdroot; %handle for the current model ("system")
      | first = get_param(sys,'Created');
      | first = first(end-3:end);  %year is last four digits
      | 
      | last = get_param(sys,'LastModifiedDate');
      | if isempty(last)
      |     last = datestr(now,'yyyy');
      | else
      |     last = last(end-3:end);
      | end
      | 
      | if strcmp(first,last)
      |     fprintf('%s -- Copyright %s Nexteer',NxtrConf,first)
      | else
      |     fprintf('%s -- %s%s- %s Nexteer',NxtrConf,char(169),first,last)
      | end
  Sts : Outport
  wires:
  Constant/1 -> Sts/1

== system ES101A_DiagcMgr/DiagcMgr/GetNtcQlfrStsCore /SIGQLFR_FAILD ==
  Action Port : ActionPort  ActionType=else
  Passd : Constant  Value=2  OutDataTypeStr=uint8
  NtcQlfr : Outport  InitialOutput=2
  wires:
  Passd/1 -> NtcQlfr/1

== system ES101A_DiagcMgr/DiagcMgr/GetNtcQlfrStsCore /SIGQLFR_NORES ==
  Action Port : ActionPort  ActionType=then
  NoRes : Constant  Value=0  OutDataTypeStr=uint8
  NtcQlfr : Outport  InitialOutput=0
  wires:
  NoRes/1 -> NtcQlfr/1

== system ES101A_DiagcMgr/DiagcMgr/GetNtcQlfrStsCore /SIGQLFR_PASSD ==
  Action Port : ActionPort  ActionType=elseif
  Passd : Constant  OutDataTypeStr=uint8
  NtcQlfr : Outport  InitialOutput=1
  wires:
  Passd/1 -> NtcQlfr/1

== system ES101A_DiagcMgr/DiagcMgr/GetNtcStsCore/CopyRight2 ==

== system ES101A_DiagcMgr/DiagcMgr/GetNtcStsCore/GetNtcInfoAppIX ==
  NtcInfoIdx_ArgIn : Inport
  Action Port : ActionPort  ActionType=case
  CopyRight2 : Subsystem  Description=|  mask(Copyright Information){none=on}
      | Copyright info block.                                               
      |                                                                     
      | Place copyright information at the top of every subsystem in design.
      mask prompts: none "No parameters"
      mask help: Place copyright information at the top of every subsystem in design.
      mask Display:
      | NxtrConf = 'Nexteer Confidential';
      | 
      | sys = bdroot; %handle for the current model ("system")
      | first = get_param(sys,'Created');
      | first = first(end-3:end);  %year is last four digits
      | 
      | last = get_param(sys,'LastModifiedDate');
      | if isempty(last)
      |     last = datestr(now,'yyyy');
      | else
      |     last = last(end-3:end);
      | end
      | 
      | if strcmp(first,last)
      |     fprintf('%s -- Copyright %s Nexteer',NxtrConf,first)
      | else
      |     fprintf('%s -- %s%s- %s Nexteer',NxtrConf,char(169),first,last)
      | end
  Data Store Read : DataStoreRead  DataStoreName=DiagcMgrNtcInfoX
  Selector : Selector  IndexMode=Zero-based  InputPortWidth=14  IndexOptions=Index vector (port)  Indices=[1 3]  OutputSizes=1
  NtcInfo_ArgOut : Outport
  wires:
  Data Store Read/1 -> Selector/1
  NtcInfoIdx_ArgIn/1 -> Selector/2
  Selector/1 -> NtcInfo_ArgOut/1

== system ES101A_DiagcMgr/DiagcMgr/GetNtcStsCore/NTC Default Status ==
  Action Port : ActionPort  ActionType=default
  Constant : Constant  Value=DIAGCMGR_NTCINFOSTSTESTNOTCMPLTHISIGNCYC_CNT_U08  OutDataTypeStr=uint8
  CopyRight2 : Subsystem  Description=|  mask(Copyright Information){none=on}
      | Copyright info block.                                               
      |                                                                     
      | Place copyright information at the top of every subsystem in design.
      mask prompts: none "No parameters"
      mask help: Place copyright information at the top of every subsystem in design.
      mask Display:
      | NxtrConf = 'Nexteer Confidential';
      | 
      | sys = bdroot; %handle for the current model ("system")
      | first = get_param(sys,'Created');
      | first = first(end-3:end);  %year is last four digits
      | 
      | last = get_param(sys,'LastModifiedDate');
      | if isempty(last)
      |     last = datestr(now,'yyyy');
      | else
      |     last = last(end-3:end);
      | end
      | 
      | if strcmp(first,last)
      |     fprintf('%s -- Copyright %s Nexteer',NxtrConf,first)
      | else
      |     fprintf('%s -- %s%s- %s Nexteer',NxtrConf,char(169),first,last)
      | end
  Sts : Outport
  wires:
  Constant/1 -> Sts/1

== system ES101A_DiagcMgr/DiagcMgr/ReadNtcFltAry/CopyRight1 ==

== system ES101A_DiagcMgr/DiagcMgr/ReadNtcFltAry/Initialize NtcMapIdx Clear HistReadFltAryIdx, ReadFltAryIdx and HistReadFltAryTempIdx ==
  CopyRight2 : Subsystem  Description=|  mask(Copyright Information){none=on}
      | Copyright info block.                                               
      |                                                                     
      | Place copyright information at the top of every subsystem in design.
      mask prompts: none "No parameters"
      mask help: Place copyright information at the top of every subsystem in design.
      mask Display:
      | NxtrConf = 'Nexteer Confidential';
      | 
      | sys = bdroot; %handle for the current model ("system")
      | first = get_param(sys,'Created');
      | first = first(end-3:end);  %year is last four digits
      | 
      | last = get_param(sys,'LastModifiedDate');
      | if isempty(last)
      |     last = datestr(now,'yyyy');
      | else
      |     last = last(end-3:end);
      | end
      | 
      | if strcmp(first,last)
      |     fprintf('%s -- Copyright %s Nexteer',NxtrConf,first)
      | else
      |     fprintf('%s -- %s%s- %s Nexteer',NxtrConf,char(169),first,last)
      | end
  Data Store Write2 : DataStoreWrite  DataStoreName=NtcMapIdx
  Data Store Write3 : DataStoreWrite  DataStoreName=ReadFltInfoIdx
  Data Store Write4 : DataStoreWrite  DataStoreName=HistReadFltAryIdx
  Data Store Write5 : DataStoreWrite  DataStoreName=HistReadFltAryTempIdx
  Initial Value : Constant  OutDataTypeStr=uint8
  Initial Value1 : Constant  Value=0  OutDataTypeStr=uint8
  Initial Value2 : Constant  Value=0  OutDataTypeStr=uint8
  Initial Value3 : Constant  Value=0  OutDataTypeStr=uint8
  wires:
  Initial Value/1 -> Data Store Write2/1
  Initial Value1/1 -> Data Store Write3/1
  Initial Value2/1 -> Data Store Write4/1
  Initial Value3/1 -> Data Store Write5/1

== system ES101A_DiagcMgr/DiagcMgr/ReadNtcFltAry/Send out data ==
  CopyRight2 : Subsystem  Description=|  mask(Copyright Information){none=on}
      | Copyright info block.                                               
      |                                                                     
      | Place copyright information at the top of every subsystem in design.
      mask prompts: none "No parameters"
      mask help: Place copyright information at the top of every subsystem in design.
      mask Display:
      | NxtrConf = 'Nexteer Confidential';
      | 
      | sys = bdroot; %handle for the current model ("system")
      | first = get_param(sys,'Created');
      | first = first(end-3:end);  %year is last four digits
      | 
      | last = get_param(sys,'LastModifiedDate');
      | if isempty(last)
      |     last = datestr(now,'yyyy');
      | else
      |     last = last(end-3:end);
      | end
      | 
      | if strcmp(first,last)
      |     fprintf('%s -- Copyright %s Nexteer',NxtrConf,first)
      | else
      |     fprintf('%s -- %s%s- %s Nexteer',NxtrConf,char(169),first,last)
      | end
  Data Store Read : DataStoreRead  DataStoreName=DiagcMgrReadFltInfoAry
  DiagcMgrReadFltInfo_ArgOut : Outport
  wires:
  Data Store Read/1 -> DiagcMgrReadFltInfo_ArgOut/1
